simulink model "arduino_serial_comentado_2021_slx_realimentacion_integral"  (R2023b)
settings: Solver=VariableStepAuto  StartTime=0.0  StopTime=Inf  RelTol=1e-3
values from neighbouring files (symbols this model uses):
  A = [0 1.0000 0 0; 0 -9.3820 -30.0000 0; 0 0 0 1.0000; 0 0 -102.4000 -20.0000]    [observador.m]    (also in observador_reformulado.m = [ 0    1.0000         0         0; realimentacion.m = [ 0    1.0000         0         0; realimentacion_integral.m = [ 0    1.0000         0         0; realimentacion_integral_reformulado.m = [ 0    1.0000         0         0)
  B = [0; 0; 0; 48.5000]    [observador.m]    (also in observador_reformulado.m = [  0; realimentacion.m = [  0; realimentacion_integral.m = [  0; realimentacion_integral_reformulado.m = [  0)
  C2 = [0 0 1 0]    [realimentacion_integral.m]    (also in realimentacion_integral_reformulado.m)
  H = -Ki(end)    [realimentacion_integral.m]    (also in realimentacion_integral_reformulado.m)
  K = place(Ad,Bd,[exp(T*(k*(-10))) exp(T*(k*(-11))) exp(T*(k*(-12))) exp(T*(k*(-13)))])    [realimentacion.m]    (also in realimentacion_integral.m = -Ki(1:end-1); realimentacion_integral_reformulado.m = -Ki(1:end-1); realimentacion_referencia.m; workspace.mat = 47.2)
libraries: instrumentseriallib x2
settings Model: Creator=Claudio  LastModifiedBy=Zoe
settings DebuggingCC: UnconnectedInputMsg=warning  UnconnectedOutputMsg=warning  UnconnectedLineMsg=warning
settings ModelReferenceCC: EnableRefExpFcnMdlSchedulingChecks=on
settings RTWCC: DLArmComputeVersion=19.05

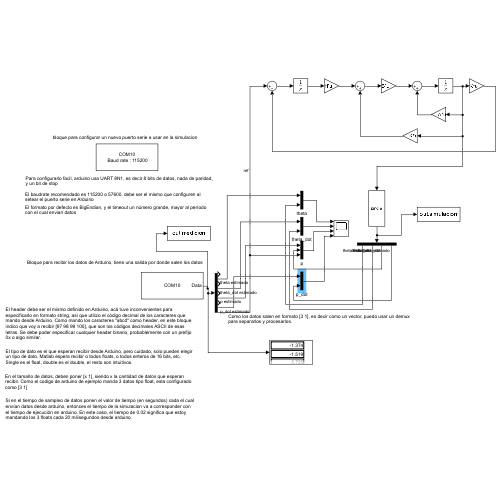
[thumbnail: Simulink's stored preview of the top-level diagram]
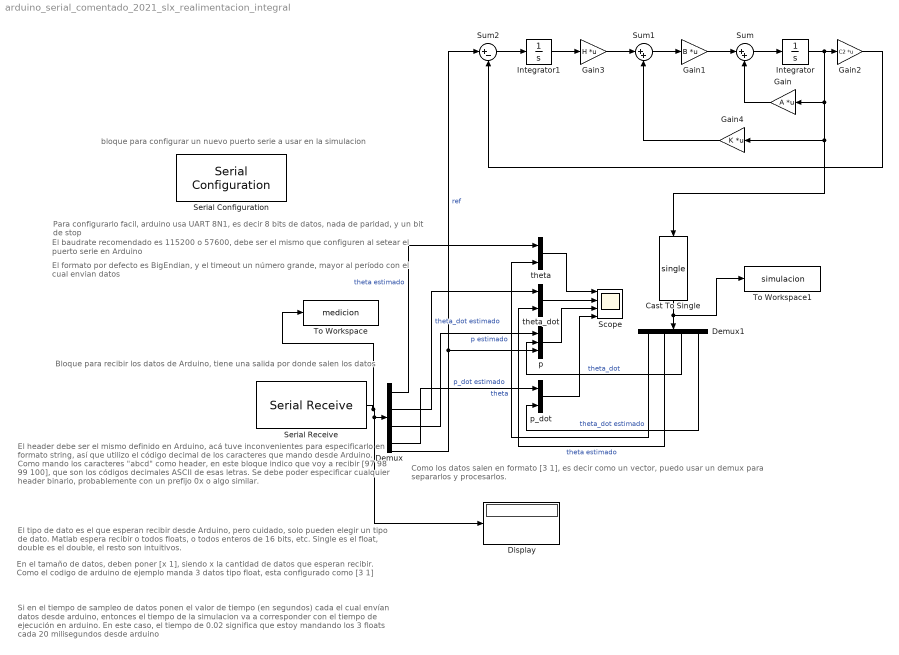
== system arduino_serial_comentado_2021_slx_realimentacion_integral ==
  note: Como los datos salen en formato [3 1], es decir como un vector, puedo usar un demux para separarlos y procesarlos.
  note: Si en el tiempo de sampleo de datos ponen el valor de tiempo (en segundos) cada el cual envían datos desde arduino, entonces el tiempo de la simulacion va a corresponder con el tiempo de ejecución en arduino. En este caso, el tiempo de 0.02 significa que estoy mandando los 3 floats cada 20 milisegundos desde arduino
  note: En el tamaño de datos, deben poner [x 1], siendo x la cantidad de datos que esperan recibir. Como el codigo de arduino de ejemplo manda 3 datos tipo float, esta configurado como [3 1]
  note: El tipo de dato es el que esperan recibir desde Arduino, pero cuidado, solo pueden elegir un tipo de dato. Matlab espera recibir o todos floats, o todos enteros de 16 bits, etc. Single es el float, double es el double, el resto son intuitivos.
  note: El header debe ser el mismo definido en Arduino, acá tuve inconvenientes para especificarlo en formato string, así que utilizo el código decimal de los caracteres que mando desde Arduino. Como mando los caracteres "abcd" como header, en este bloque indico que voy a recibir [97 98 99 100], que son los códigos decimales ASCII de esas letras. Se debe poder especificar cualquier header binario, probablemente con un prefijo 0x o algo similar.
  note: Bloque para recibir los datos de Arduino, tiene una salida por donde salen los datos
  note: El formato por defecto es BigEndian, y el timeout un número grande, mayor al período con el cual envian datos
  note: El baudrate recomendado es 115200 o 57600, debe ser el mismo que configuren al setear el puerto serie en Arduino
  note: Para configurarlo facil, arduino usa UART 8N1, es decir 8 bits de datos, nada de paridad, y un bit de stop
  note: bloque para configurar un nuevo puerto serie a usar en la simulacion
  Cast To Single : DataTypeConversion  OutDataTypeStr=single  SaturateOnIntegerOverflow=off  RndMeth=Floor
  Demux : Demux  Outputs=9
  Demux1 : Demux
  Display : Display
  Gain : Gain  Gain=A  Multiplication=Matrix(K*u)
  Gain1 : Gain  Gain=B  Multiplication=Matrix(K*u)
  Gain2 : Gain  Gain=C2  Multiplication=Matrix(K*u)
  Gain3 : Gain  Gain=H  Multiplication=Matrix(K*u)
  Gain4 : Gain  Gain=K  Multiplication=Matrix(K*u)
  Integrator : Integrator  InitialCondition=[0; 0; 0; 0]
  Integrator1 : Integrator
  Scope : Scope  NumInputPorts=4
  Serial Configuration : instrumentseriallib/Serial Configuration  Priority=-200000  PortSel=COM10  Port=COM10  ComPort=COM10  BaudRate=115200  DataBits=8  Parity=none  StopBits=1  ByteOrder=big-endian  FlowControl=none  Timeout=10  SimulateUsing=Interpreted execution  BlockInModel=on  aMode=1
  Serial Receive : instrumentseriallib/Serial Receive  Priority=1  PortSel=COM10  Port=COM10  ComPort=COM10  DataType=single  SaveDataType=uint8  ToggleHeader=on  Header="[ 97   98   99  100 ]"  ToggleTerminator=off  Terminator=<none>  CustomTerminator=[]  InputFormat=Column major  ToggleDataSize=on  DataSize=[9 1]  EnableBlockingMode=on  ActionDataUnavailable=Output last received value  ActionWhenDataUnavailable=Output last received value  CustomValue=0  SampleTime=0.02  SimulateUsing=Interpreted execution  BlockInModel=on  aMode=1
  Sum : Sum  Inputs=|++
  Sum1 : Sum  Inputs=|++
  Sum2 : Sum  Inputs=|+-
  To Workspace : ToWorkspace  VariableName=medicion  SaveFormat=Timeseries  SampleTime=-1
  To Workspace1 : ToWorkspace  VariableName=simulacion  SaveFormat=Timeseries  SampleTime=-1
  p : Mux  Inputs=3
  p_dot : Mux  Inputs=2
  theta : Mux  Inputs=2
  theta_dot : Mux  Inputs=2
  wires:
  Serial Receive/1 -> To Workspace/1, Display/1, Demux/1
  Demux/2 -> theta/1  "theta estimado"
  Demux/4 -> theta_dot/1  "theta_dot estimado"
  Demux/6 -> p/1  "p estimado"
  p/1 -> Scope/3
  theta_dot/1 -> Scope/2
  theta/1 -> Scope/1
  p_dot/1 -> Scope/4
  Demux/8 -> p_dot/1  "p_dot estimado"
  Gain1/1 -> Sum/1
  Integrator/1 -> Gain4/1, Cast To Single/1, Gain/1, Gain2/1
  Gain/1 -> Sum/2
  Demux/9 -> p/3, Sum2/1  "ref"
  Demux1/1 -> theta/2  "theta"
  Demux1/2 -> theta_dot/2  "theta estimado"
  Cast To Single/1 -> Demux1/1, To Workspace1/1
  Demux1/3 -> p/2  "theta_dot"
  Demux1/4 -> p_dot/2  "theta_dot estimado"
  Sum1/1 -> Gain1/1
  Integrator1/1 -> Gain3/1
  Sum2/1 -> Integrator1/1
  Gain4/1 -> Sum1/2
  Sum/1 -> Integrator/1
  Gain3/1 -> Sum1/1
  Gain2/1 -> Sum2/2
